simulink model "sistema_electrico"  (R2018a)
settings: Solver=VariableStepAuto  StartTime=0.0  StopTime=0.012  MaxStep=1e-5  RelTol=1e-3
values from neighbouring files (symbols this model uses):
  A = [0 1 0 0 0 0 ... (first row only)    [Problem_5_Matlab.m]    (also in anexo_parcial.m = [-R/L 0 -ke/L 0 0; ejemplo_electrico.m = [0 -1/L; 1/C -1/(R*C)]; ejemplo_mecanico.m = [0 1 0 0; ejercicio7_taller2SM.m = [0 1; -(K2+K1/R^2)/(M+J/R^2) -b/(M+J/R^2)])
  B = [0 0 ... (first row only)    [Problem_5_Matlab.m]    (also in anexo_parcial.m = [1/L 0 0 0 0]'; ejemplo_electrico.m = [1/L; 0]; ejemplo_mecanico.m = [0; 1/M1;0 ;0]; ejercicio7_taller2SM.m = [0 1/(M+J/R^2)]')
  C = [K1/(J2+M*r^2) 0 -(K1+K2*r^2)/(J2+M*r^2) -(D3+fv*r^2)/(J2+M*r^2) 0 D3/(J2+M*r^2)]*r    [Problem_5_Matlab.m]    (also in anexo_parcial.m = [0 1 0 0 0]; ejemplo_electrico.m = 1e-06; ejemplo_mecanico.m = [0 0 1 0]; ejercicio7_taller2SM.m = [1 0; 1/R 0])
  C1 = [0 1]    [ejemplo_electrico.m]
  D = [0 M*r^2/(J2+M*r^2)]    [Problem_5_Matlab.m]    (also in anexo_parcial.m = []; ejemplo_electrico.m = 0; ejemplo_mecanico.m = []; ejercicio7_taller2SM.m = [])
  L = 1e-3    (= 0.001)    [anexo_parcial.m]    (also in ejemplo_electrico.m = 0.1; motord_DC_rot.m = 0.0001)
  R = 10    [anexo_parcial.m]    (also in ejemplo_electrico.m = 1000; ejercicio7_taller2SM.m = 0.01; motord_DC_rot.m; nivel_tanque.m = 37)
settings Model: Creator=carma  LastModifiedBy=carma

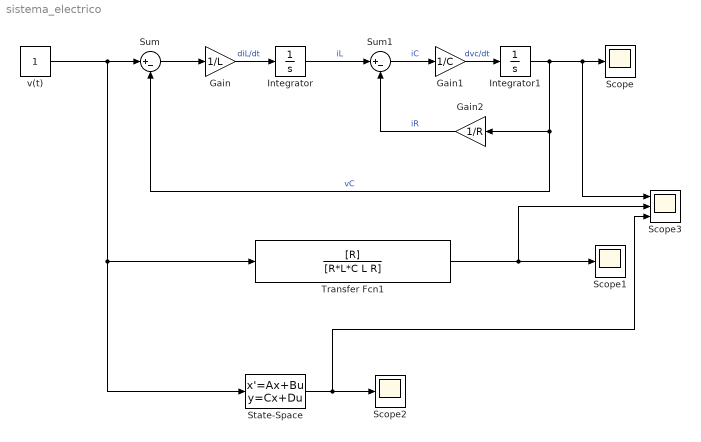
== system sistema_electrico ==
  Gain : Gain  Gain=1/L
  Gain1 : Gain  Gain=1/C
  Gain2 : Gain  Gain=1/R
  Integrator : Integrator
  Integrator1 : Integrator
  Scope : Scope
  Scope1 : Scope
  Scope2 : Scope
  Scope3 : Scope  NumInputPorts=3
  State-Space : StateSpace  A=A  B=B  C=C1  D=D  InitialCondition=0
  Sum : Sum  Inputs=|+-
  Sum1 : Sum  Inputs=|+-
  Transfer Fcn1 : TransferFcn  Numerator=[R]  Denominator=[R*L*C L R]
  v(t) : Constant
  wires:
  v(t)/1 -> State-Space/1, Transfer Fcn1/1, Sum/1
  Sum/1 -> Gain/1
  Gain/1 -> Integrator/1  "diL/dt"
  Integrator/1 -> Sum1/1  "iL"
  Gain2/1 -> Sum1/2  "iR"
  Sum1/1 -> Gain1/1  "iC"
  Gain1/1 -> Integrator1/1  "dvc/dt"
  Integrator1/1 -> Gain2/1, Sum/2, Scope3/1, Scope/1  "vC"
  Transfer Fcn1/1 -> Scope3/2, Scope1/1
  State-Space/1 -> Scope3/3, Scope2/1
